simulink model "elec443_lab"  (R2025b)
settings: Solver=ode1  StartTime=0.0  StopTime=20  FixedStep=0.002  RelTol=1e-3  EnableMultiTasking=on
values from neighbouring files (symbols this model uses):
  K = 8.35    [elec443_lab1_setup.m]
  K_CABLE = 1    [elec443_lab1_setup.m]
  K_ENC = 0    [config_srv02.m]
  tau = 0.03478    [elec443_lab1_setup.m]
  VMAX_DAC = 10    [elec443_lab1_setup.m]
  VMAX_UPM = 0    [config_srv02.m]
  wcf_e = 2 * pi * 25.0    (= 157.079632679)    [elec443_lab1_setup.m]
  zetaf_e = 0.9    [elec443_lab1_setup.m]
undefined symbols (not defined in the file or in its folder): HIL
libraries: quarc_library x3, simulink x2
settings Model: SimulationMode=external  ExtModeTrigDuration=1000000  Creator=6ah19  LastModifiedBy=noahw
settings SolverCC: AlgebraicLoopSolver=TrustRegion  PositivePriorityOrder=on
settings DataIOCC: LimitDataPoints=on  SaveFormat=Array  SignalLoggingSaveFormat=ModelDataLogs  ReturnWorkspaceOutputs=off
settings OptimizationCC: ExpressionDepthLimit=2147483647.0
settings DebuggingCC: UnderspecifiedInitializationDetection=Classic  MergeDetectMultiDrivingBlocksExec=none  SolverPrmCheckMsg=warning  FcnCallInpInsideContextMsg=warning  UnconnectedInputMsg=warning  UnconnectedOutputMsg=warning  UnconnectedLineMsg=warning  StateNameClashWarn=warning  SFUnexpectedBacktrackingDiag=warning  SFNoUnconditionalDefaultTransitionDiag=warning  SFExecutionAtInitializationDiag=none  ArithmeticOperatorsInVariantConditions=warning
settings ModelReferenceCC: EnableRefExpFcnMdlSchedulingChecks=on  PropagateSignalLabelsOutOfModel=off
settings SFSimCC: SimUseLocalCustomCode=off  CustomCodeUndefinedFunction=UseInterfaceOnly
settings RTWCC: SystemTargetFile=quarc_win64.tlc  TemplateMakefile=quarc_default_tmf  RTWUseLocalCustomCode=off  Toolchain=QUARC win64 | nmake (64-bit Windows)  BuildConfiguration=Faster Runs  GPUComputeCapability=3.5  Description=QUARC Win64 Target Using Toolchain
settings CodeAppCC: StateflowObjectComments=on
settings STFCustomTargetCC: SystemTargetFile=quarc_win64.tlc  UseToolchainInfoCompliant=on  StopOnOverrun=off
settings GRTTargetCC: ExtMode=on  ExtModeMexFile=quarc_comm  TargetLangStandard=C89/C90 (ANSI)  ParMdlRefBuildCompliant=off  CompOptLevelCompliant=off  CombineOutputUpdateFcns=off  MatFileLogging=off  CPPClassGenCompliant=off  GRTInterface=on
settings ConfigComp: CovMetricSettings=dw  CovSaveCumulativeToWorkspaceVar=on  CovSaveSingleToWorkspaceVar=on  CovExternalEMLEnable=off

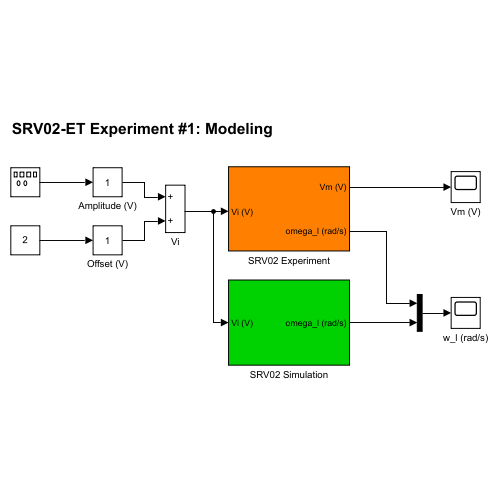
[thumbnail: Simulink's stored preview of the top-level diagram]
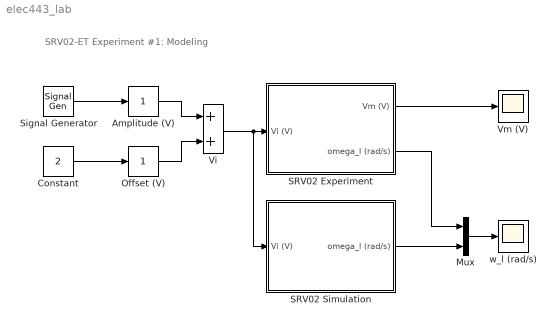
== system elec443_lab ==
  note: SRV02-ET Experiment #1: Modeling
  Amplitude (V) : simulink/Math Operations/Slider Gain  gain=1  low=0  high=10
  Constant : Constant  Value=2
  Mux : Mux  Inputs=2
  Offset (V) : simulink/Math Operations/Slider Gain  gain=1  low=-5  high=5
  SRV02 Experiment : Subsystem
  SRV02 Simulation : Subsystem
  Signal Generator : SignalGenerator  WaveForm=square  Frequency=0.2
  Vi : Sum
  Vm (V) : Scope
      settings: ActiveDisplayYMinimum=0.75  ActiveDisplayYMaximum=3.25  DataLoggingVariableName=Vm  DataLoggingSaveFormat=Array
  w_l (rad/s) : Scope
      settings: ActiveDisplayYMinimum=-1.89218  ActiveDisplayYMaximum=27.02965  DataLoggingVariableName=wl  DataLoggingSaveFormat=Array
  wires:
  Constant/1 -> Offset (V)/1
  Offset (V)/1 -> Vi/2
  Mux/1 -> w_l (rad/s)/1
  SRV02 Experiment/1(Vm (V)) -> Vm (V)/1
  SRV02 Simulation/1(omega_l (rad/s)) -> Mux/2
  SRV02 Experiment/2(omega_l (rad/s)) -> Mux/1
  Signal Generator/1 -> Amplitude (V)/1
  Amplitude (V)/1 -> Vi/1
  Vi/1 -> SRV02 Simulation/1(Vi (V)), SRV02 Experiment/1(Vi (V))

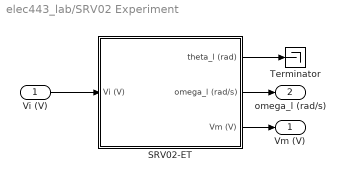
== system elec443_lab/SRV02 Experiment ==
  Vi (V) : Inport
  SRV02-ET : Subsystem
  Terminator : Terminator
  Vm (V) : Outport
  omega_l (rad/s) : Outport  Port=2
  wires:
  SRV02-ET/3(Vm (V)) -> Vm (V)/1
  Vi (V)/1 -> SRV02-ET/1(Vi (V))
  SRV02-ET/2(omega_l (rad/s)) -> omega_l (rad/s)/1
  SRV02-ET/1(theta_l (rad)) -> Terminator/1

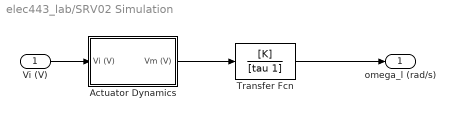
== system elec443_lab/SRV02 Simulation ==
  Vi (V) : Inport
  Actuator Dynamics : Subsystem
  Transfer Fcn : TransferFcn  Numerator=[K]  Denominator=[tau 1]
  omega_l (rad/s) : Outport
  wires:
  Vi (V)/1 -> Actuator Dynamics/1(Vi (V))
  Actuator Dynamics/1(Vm (V)) -> Transfer Fcn/1
  Transfer Fcn/1 -> omega_l (rad/s)/1

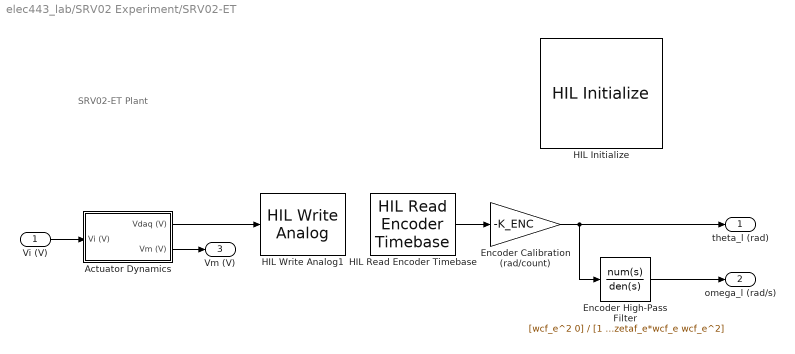
== system elec443_lab/SRV02 Experiment/SRV02-ET ==
  note: SRV02-ET Plant
  Vi (V) : Inport
  Actuator Dynamics : Subsystem
  Encoder Calibration (rad/count) : Gain  Gain=-K_ENC  SaturateOnIntegerOverflow=on  OutDataTypeStr=Inherit: Same as input  ParamDataTypeStr=Inherit: Same as input
  Encoder High-Pass Filter : TransferFcn  Numerator=[wcf_e^2 0]  Denominator=[1 2*zetaf_e*wcf_e wcf_e^2]
  HIL Initialize : quarc_library/Data Acquisition/Generic/Configuration/HIL Initialize  object_name=HIL-1  board_type=q2_usb  board_number=0  board_options=d0=digital;d1=digital;led=auto;update_rate=normal;decimation=1  exclusive=off  active=on  hardware_clocks=[0]  clock_modes=[]  initial_clock_frequencies=[]  set_clock_params_at_start=off  set_clock_params_at_switch_in=off  set_clock_frequencies_at_start=off  set_clock_frequencies_at_switch_in=off  analog_input_channels=[0:1]  analog_input_configurations=[]  analog_input_maximums=10  analog_input_minimums=-10  set_analog_input_params_at_start=on  set_analog_input_params_at_switch_in=off  analog_output_channels=[0:1]  analog_output_maximums=10  analog_output_minimums=-10  initial_analog_outputs=[0]  final_analog_outputs=[0]  watchdog_analog_outputs=0  set_analog_output_params_at_start=on  set_analog_output_params_at_switch_in=off  set_analog_outputs_at_start=on  set_analog_outputs_at_switch_in=off  set_analog_outputs_at_terminate=on  set_analog_outputs_at_switch_out=off  set_analog_outputs_on_watchdog=off  digital_input_channels=[]  digital_output_channels=[]  digital_output_configuration=[]  initial_digital_outputs=[1]  final_digital_outputs=[1]  watchdog_digital_outputs=[1]  set_digital_output_params_at_start=off  set_digital_output_params_at_switch_in=off  set_digital_outputs_at_start=on  set_digital_outputs_at_switch_in=off  set_digital_outputs_at_terminate=on  set_digital_outputs_at_switch_out=off  set_digital_outputs_on_watchdog=off  encoder_channels=[0:1]  quadrature=[4]  encoder_filter_frequency=[]  initial_encoder_counts=[0]  set_encoder_params_at_start=on  set_encoder_params_at_switch_in=off  set_encoder_counts_at_start=on  set_encoder_counts_at_switch_in=off  pwm_channels=[]  pwm_modes=[0]  pwm_frequency=1/0.020  pwm_configuration=[]  pwm_alignment=[]  pwm_polarity=[]  pwm_leading_deadband=[]  pwm_trailing_deadband=[]  initial_pwm_outputs=[0]  final_pwm_outputs=[0]  watchdog_pwm_outputs=[0]  set_pwm_params_at_start=on  set_pwm_params_at_switch_in=off  set_pwm_outputs_at_start=on  set_pwm_outputs_at_switch_in=off  set_pwm_outputs_at_terminate=on  set_pwm_outputs_at_switch_out=off  set_pwm_outputs_on_watchdog=off  other_output_channels=[]  initial_other_outputs=[]  final_other_outputs=[]  watchdog_other_outputs=[]  set_other_outputs_at_start=off  set_other_outputs_at_switch_in=off  set_other_outputs_at_terminate=off  set_other_outputs_at_switch_out=off  set_other_outputs_on_watchdog=off
  HIL Read Encoder Timebase : quarc_library/Data Acquisition/Generic/Timebases/HIL Read Encoder Timebase  object_name=HIL-1  clock=0  channels=0  active=on  vector_output=off  data_type_mode=Inherit via back propagation  data_type=double  overflow_mode=Discard on overflow  samples_in_buffer=1
  HIL Write Analog1 : quarc_library/Data Acquisition/Generic/Immediate I//O/HIL Write Analog  object_name=HIL-1  channels=0  sample_time=-1  active=on  vector_input=off
  theta_l (rad) : Outport  InitialOutput=0
  omega_l (rad/s) : Outport  Port=2  InitialOutput=0
  Vm (V) : Outport  Port=3  InitialOutput=0
  wires:
  HIL Read Encoder Timebase/1 -> Encoder Calibration (rad/count)/1
  Encoder Calibration (rad/count)/1 -> Encoder High-Pass Filter/1, theta_l (rad)/1
  Encoder High-Pass Filter/1 -> omega_l (rad/s)/1
  Actuator Dynamics/2(Vm (V)) -> Vm (V)/1
  Actuator Dynamics/1(Vdaq (V)) -> HIL Write Analog1/1
  Vi (V)/1 -> Actuator Dynamics/1(Vi (V))

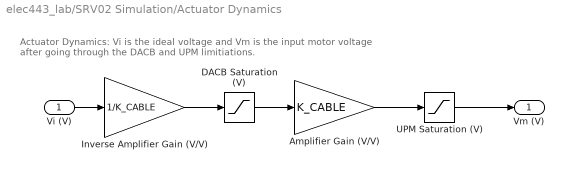
== system elec443_lab/SRV02 Simulation/Actuator Dynamics ==
  note: Actuator Dynamics: Vi is the ideal voltage and Vm is the
      | input motor voltage after going through the DACB and UPM limitiations.
  Vi (V) : Inport
  Amplifier Gain (V/V) : Gain  Gain=K_CABLE
  DACB Saturation (V) : Saturate  UpperLimit=VMAX_DAC  LowerLimit=-VMAX_DAC
  Inverse Amplifier Gain (V/V) : Gain  Gain=1/K_CABLE
  UPM Saturation (V) : Saturate  UpperLimit=VMAX_UPM  LowerLimit=-VMAX_UPM
  Vm (V) : Outport
  wires:
  Inverse Amplifier Gain (V/V)/1 -> DACB Saturation (V)/1
  DACB Saturation (V)/1 -> Amplifier Gain (V/V)/1
  Amplifier Gain (V/V)/1 -> UPM Saturation (V)/1
  Vi (V)/1 -> Inverse Amplifier Gain (V/V)/1
  UPM Saturation (V)/1 -> Vm (V)/1

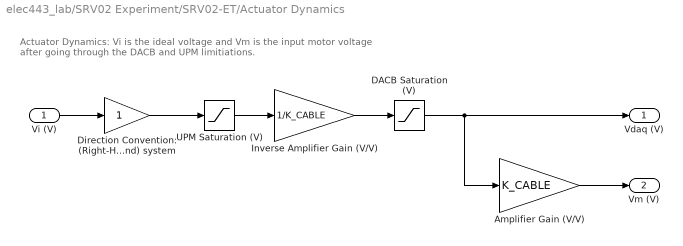
== system elec443_lab/SRV02 Experiment/SRV02-ET/Actuator Dynamics ==
  note: Actuator Dynamics: Vi is the ideal voltage and Vm is the
      | input motor voltage after going through the DACB and UPM limitiations.
  Vi (V) : Inport
  Amplifier Gain (V/V) : Gain  Gain=K_CABLE
  DACB Saturation (V) : Saturate  UpperLimit=VMAX_DAC  LowerLimit=-VMAX_DAC
  Direction Convention: (Right-Hand) system : Gain  SaturateOnIntegerOverflow=on  OutDataTypeStr=Inherit: Same as input  ParamDataTypeStr=Inherit: Same as input
  Inverse Amplifier Gain (V/V) : Gain  Gain=1/K_CABLE
  UPM Saturation (V) : Saturate  UpperLimit=VMAX_UPM  LowerLimit=-VMAX_UPM
  Vdaq (V) : Outport
  Vm (V) : Outport  Port=2
  wires:
  Direction Convention: (Right-Hand) system/1 -> UPM Saturation (V)/1
  Amplifier Gain (V/V)/1 -> Vm (V)/1
  DACB Saturation (V)/1 -> Vdaq (V)/1, Amplifier Gain (V/V)/1
  Inverse Amplifier Gain (V/V)/1 -> DACB Saturation (V)/1
  UPM Saturation (V)/1 -> Inverse Amplifier Gain (V/V)/1
  Vi (V)/1 -> Direction Convention: (Right-Hand) system/1
